simulink model "sim_DiscMRE_case1"  (R2024a)
settings: Solver=ode1  StartTime=0.0  StopTime=150  FixedStep=Ts  MaxStep=Ts  RelTol=1e-4
values from neighbouring files (symbols this model uses):
  x0 = x_init    [TO_sys.m]
undefined symbols (not defined in the file or in its folder): b0, b1, c1, c2, c3, curN, gamma, kpa, N, Phi0, th, Ts, vari, z0, zeta0
libraries: matrix_library x2
settings Model: Creator=stt  LastModifiedBy=stt
settings SolverCC: SolverResetMethod=Robust
settings OptimizationCC: ReuseModelBlockBuffer=off
settings RTWCC: GPUComputeCapability=3.5

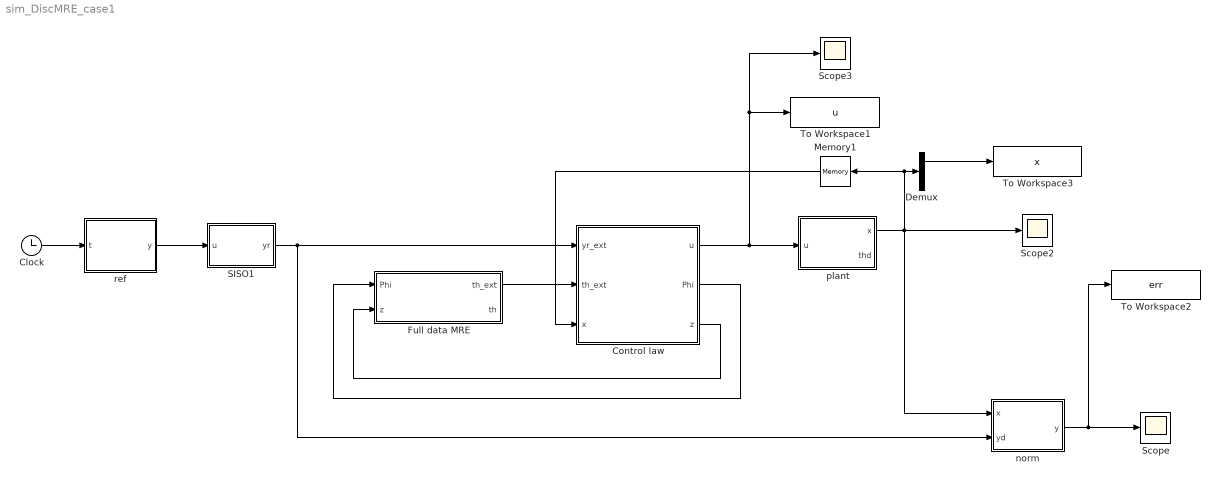
== system sim_DiscMRE_case1 ==
  Clock : Clock
  Control law : Subsystem
  Demux : Demux  Outputs=3
  Full data MRE : Subsystem
  Memory1 : Memory  InitialCondition=x0
  SISO1 : Subsystem
  Scope : Scope
  Scope2 : Scope
  Scope3 : Scope
  To Workspace1 : ToWorkspace  VariableName=u  SaveFormat=Timeseries  SampleTime=-1
  To Workspace2 : ToWorkspace  VariableName=err  SaveFormat=Timeseries  SampleTime=-1
  To Workspace3 : ToWorkspace  VariableName=x  SaveFormat=Timeseries  SampleTime=-1
  norm : MATLAB Function  TreatAsAtomicUnit=on
  plant : Subsystem
  ref : MATLAB Function  TreatAsAtomicUnit=on
  wires:
  SISO1/1(yr) -> norm/2(yd), Control law/1(yr_ext)
  norm/1(y) -> To Workspace2/1, Scope/1
  plant/1(x) -> Demux/1, Memory1/1, norm/1(x), Scope2/1
  Demux/1 -> To Workspace3/1
  Clock/1 -> ref/1(t)
  Control law/2(Phi) -> Full data MRE/1(Phi)
  Control law/1(u) -> To Workspace1/1, Scope3/1, plant/1(u)
  Memory1/1 -> Control law/3(x)
  Full data MRE/1(th_ext) -> Control law/2(th_ext)
  Control law/3(z) -> Full data MRE/2(z)
  ref/1(y) -> SISO1/1(u)

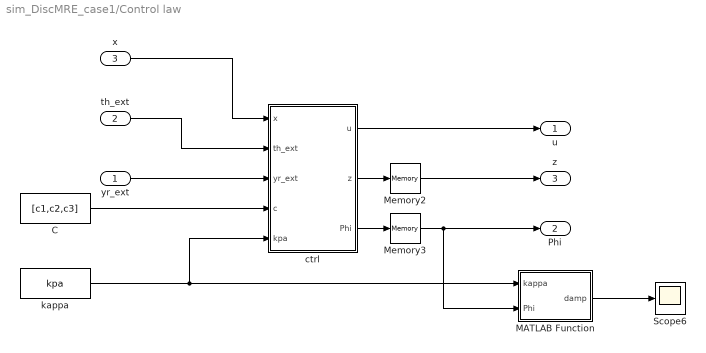
== system sim_DiscMRE_case1/Control law ==
  yr_ext : Inport
  th_ext : Inport  Port=2
  x : Inport  Port=3
  C : Constant  Value=[c1,c2,c3]
  MATLAB Function : MATLAB Function  TreatAsAtomicUnit=on
  Memory2 : Memory  InitialCondition=z0
  Memory3 : Memory  InitialCondition=Phi0
  Scope6 : Scope
  ctrl : MATLAB Function  TreatAsAtomicUnit=on
  kappa : Constant  Value=kpa
  u : Outport
  Phi : Outport  Port=2
  z : Outport  Port=3
  wires:
  ctrl/3(Phi) -> Memory3/1
  Memory3/1 -> MATLAB Function/2(Phi), Phi/1
  th_ext/1 -> ctrl/2(th_ext)
  kappa/1 -> ctrl/5(kpa), MATLAB Function/1(kappa)
  C/1 -> ctrl/4(c)
  Memory2/1 -> z/1
  ctrl/2(z) -> Memory2/1
  yr_ext/1 -> ctrl/3(yr_ext)
  x/1 -> ctrl/1(x)
  ctrl/1(u) -> u/1
  MATLAB Function/1(damp) -> Scope6/1

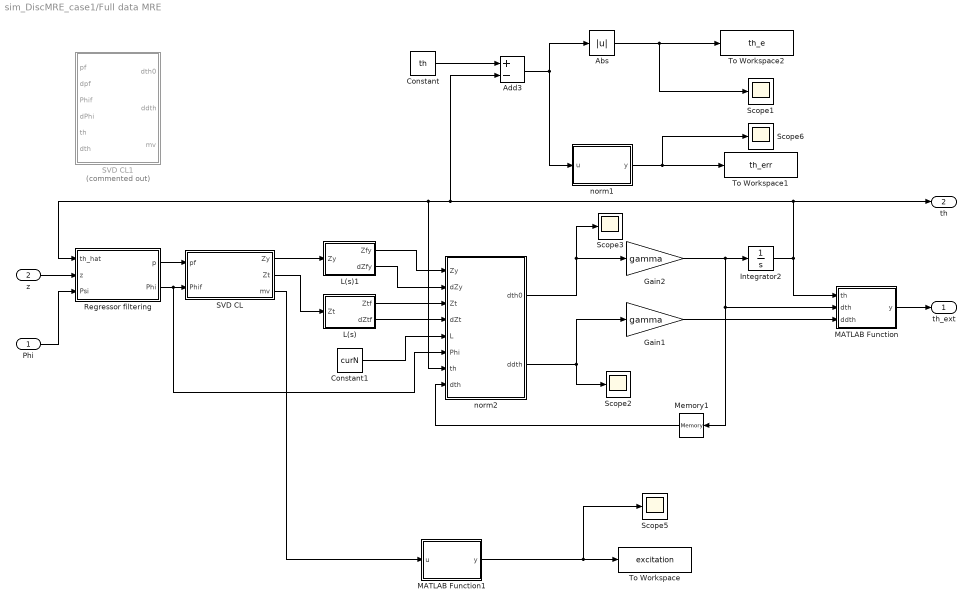
== system sim_DiscMRE_case1/Full data MRE ==
  Phi : Inport
  z : Inport  Port=2
  Abs : Abs  SaturateOnIntegerOverflow=off
  Add3 : Sum  Inputs=+-
  Constant : Constant  Value=th
  Constant1 : Constant  Value=curN
  Gain1 : Gain  Gain=gamma
  Gain2 : Gain  Gain=gamma
  Integrator2 : Integrator  InitialCondition=zeros(N,1)
  L(s) : Subsystem
  L(s)1 : Subsystem
  MATLAB Function : MATLAB Function  TreatAsAtomicUnit=on
  MATLAB Function1 : MATLAB Function  TreatAsAtomicUnit=on
  Memory1 : Memory  InitialCondition=zeros(N,1)
  Regressor filtering : Subsystem
  SVD CL : Subsystem
  SVD CL1 : Subsystem  Commented=on
  Scope{1..3,5..6} (5 alike) : Scope
  To Workspace : ToWorkspace  VariableName=excitation  SaveFormat=Timeseries  SampleTime=-1
  To Workspace1 : ToWorkspace  VariableName=th_err  SaveFormat=Timeseries  SampleTime=-1
  To Workspace2 : ToWorkspace  VariableName=th_e  SaveFormat=Timeseries  SampleTime=-1
  norm1 : MATLAB Function  TreatAsAtomicUnit=on
  norm2 : MATLAB Function  TreatAsAtomicUnit=on
  th_ext : Outport
  th : Outport  Port=2
  wires:
  MATLAB Function/1(y) -> th_ext/1
  MATLAB Function1/1(y) -> Scope5/1, To Workspace/1
  norm1/1(y) -> To Workspace1/1, Scope6/1
  Constant/1 -> Add3/1
  z/1 -> Regressor filtering/2(z)
  Phi/1 -> Regressor filtering/3(Psi)
  Gain1/1 -> MATLAB Function/3(ddth)
  Integrator2/1 -> MATLAB Function/1(th), th/1, norm2/7(th), Regressor filtering/1(th_hat), Add3/2
  Add3/1 -> norm1/1(u), Abs/1
  Abs/1 -> To Workspace2/1, Scope1/1
  Gain2/1 -> Memory1/1, MATLAB Function/2(dth), Integrator2/1
  Regressor filtering/1(p) -> SVD CL/1(pf)
  Regressor filtering/2(Phi) -> norm2/6(Phi), SVD CL/2(Phif)
  SVD CL/3(mv) -> MATLAB Function1/1(u)
  SVD CL/1(Zy) -> L(s)1/1(Zy)
  SVD CL/2(Zt) -> L(s)/1(Zt)
  L(s)1/1(Zfy) -> norm2/1(Zy)
  L(s)1/2(dZfy) -> norm2/2(dZy)
  L(s)/1(Ztf) -> norm2/3(Zt)
  L(s)/2(dZtf) -> norm2/4(dZt)
  Constant1/1 -> norm2/5(L)
  Memory1/1 -> norm2/8(dth)
  norm2/2(ddth) -> Gain1/1, Scope2/1
  norm2/1(dth0) -> Scope3/1, Gain2/1

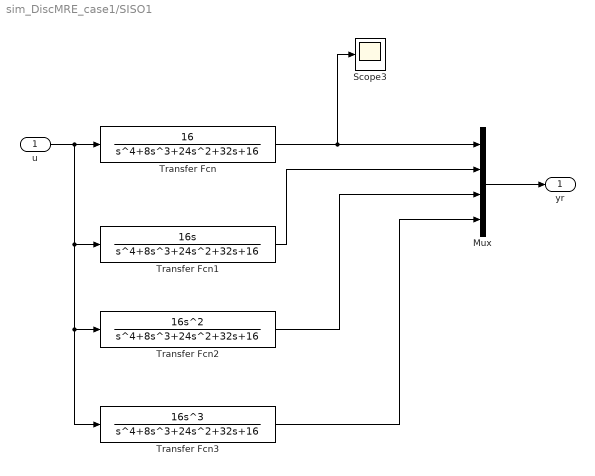
== system sim_DiscMRE_case1/SISO1 ==
  u : Inport
  Mux : Mux
  Scope3 : Scope
  Transfer Fcn : TransferFcn  Numerator=[16]  Denominator=[1 8 24 32 16]
  Transfer Fcn1 : TransferFcn  Numerator=[16 0]  Denominator=[1 8 24 32 16]
  Transfer Fcn2 : TransferFcn  Numerator=[16 0 0]  Denominator=[1 8 24 32 16]
  Transfer Fcn3 : TransferFcn  Numerator=[16 0 0 0]  Denominator=[1 8 24 32 16]
  yr : Outport
  wires:
  u/1 -> Transfer Fcn3/1, Transfer Fcn2/1, Transfer Fcn1/1, Transfer Fcn/1
  Transfer Fcn/1 -> Scope3/1, Mux/1
  Transfer Fcn1/1 -> Mux/2
  Transfer Fcn2/1 -> Mux/3
  Transfer Fcn3/1 -> Mux/4
  Mux/1 -> yr/1

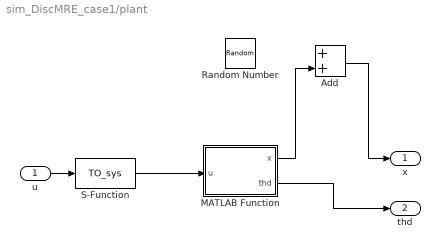
== system sim_DiscMRE_case1/plant ==
  u : Inport
  Add : Sum
  MATLAB Function : MATLAB Function  TreatAsAtomicUnit=on
  Random Number : RandomNumber  Variance=vari  SampleTime=Ts
  S-Function : S-Function  FunctionName=TO_sys  Parameters=x0,th  SFunctionDeploymentMode=off  EnableBusSupport=off
  x : Outport
  thd : Outport  Port=2
  wires:
  u/1 -> S-Function/1
  S-Function/1 -> MATLAB Function/1(u)
  Add/1 -> x/1
  MATLAB Function/2(thd) -> thd/1
  MATLAB Function/1(x) -> Add/2

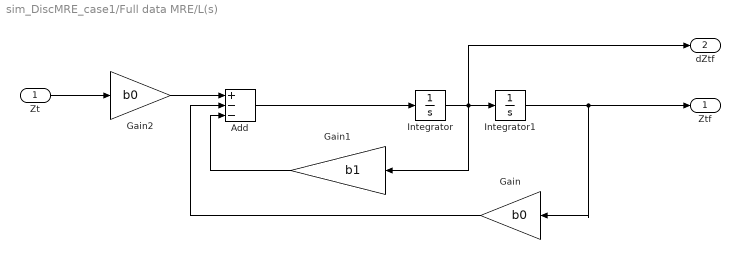
== system sim_DiscMRE_case1/Full data MRE/L(s) ==
  Zt : Inport
  Add : Sum  Inputs=+--
  Gain : Gain  Gain=b0
  Gain1 : Gain  Gain=b1
  Gain2 : Gain  Gain=b0
  Integrator : Integrator
  Integrator1 : Integrator
  Ztf : Outport
  dZtf : Outport  Port=2
  wires:
  Zt/1 -> Gain2/1
  Integrator1/1 -> Gain/1, Ztf/1
  Add/1 -> Integrator/1
  Integrator/1 -> Gain1/1, dZtf/1, Integrator1/1
  Gain1/1 -> Add/3
  Gain/1 -> Add/2
  Gain2/1 -> Add/1

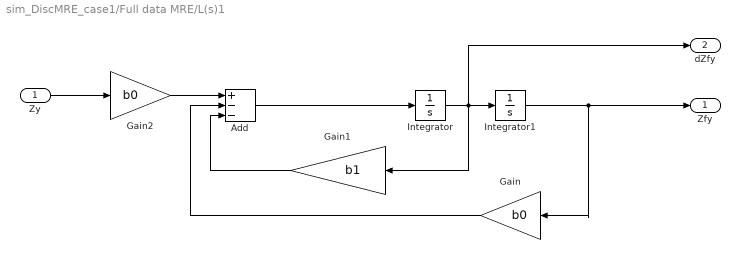
== system sim_DiscMRE_case1/Full data MRE/L(s)1 ==
  Zy : Inport
  Add : Sum  Inputs=+--
  Gain : Gain  Gain=b0
  Gain1 : Gain  Gain=b1
  Gain2 : Gain  Gain=b0
  Integrator : Integrator
  Integrator1 : Integrator
  Zfy : Outport
  dZfy : Outport  Port=2
  wires:
  Zy/1 -> Gain2/1
  Integrator1/1 -> Gain/1, Zfy/1
  Add/1 -> Integrator/1
  Integrator/1 -> Gain1/1, dZfy/1, Integrator1/1
  Gain1/1 -> Add/3
  Gain/1 -> Add/2
  Gain2/1 -> Add/1

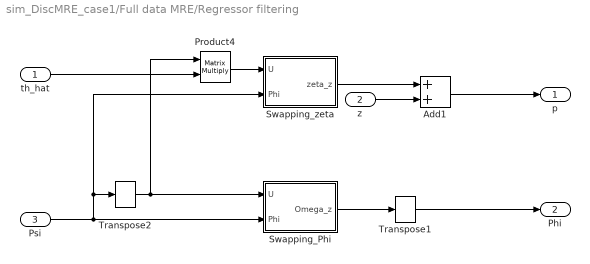
== system sim_DiscMRE_case1/Full data MRE/Regressor filtering ==
  th_hat : Inport
  z : Inport  Port=2
  Psi : Inport  Port=3
  Add1 : Sum
  Product4 : Product  Multiplication=Matrix(*)
  Swapping_Phi : Subsystem
  Swapping_zeta : Subsystem
  Transpose1 : matrix_library/Transpose
  Transpose2 : matrix_library/Transpose
  p : Outport
  Phi : Outport  Port=2
  wires:
  Product4/1 -> Swapping_zeta/1(U)
  th_hat/1 -> Product4/2
  Psi/1 -> Swapping_Phi/2(Phi), Swapping_zeta/2(Phi), Transpose2/1
  Swapping_zeta/1(zeta_z) -> Add1/1
  Transpose2/1 -> Swapping_Phi/1(U), Product4/1
  z/1 -> Add1/2
  Add1/1 -> p/1
  Swapping_Phi/1(Omega_z) -> Transpose1/1
  Transpose1/1 -> Phi/1

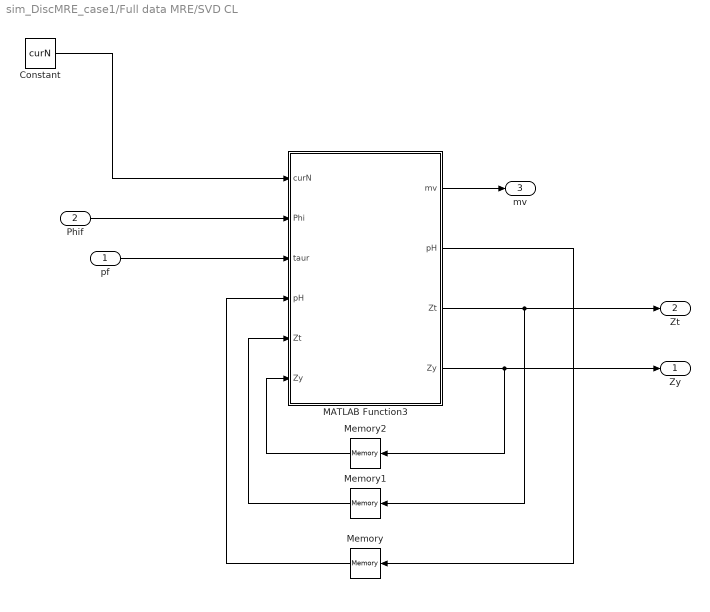
== system sim_DiscMRE_case1/Full data MRE/SVD CL ==
  pf : Inport
  Phif : Inport  Port=2
  Constant : Constant  Value=curN
  MATLAB Function3 : MATLAB Function  TreatAsAtomicUnit=on
  Memory : Memory
  Memory1 : Memory  InitialCondition=zeros(N,3*curN)
  Memory2 : Memory  InitialCondition=zeros(3*curN,1)
  Zy : Outport
  Zt : Outport  Port=2
  mv : Outport  Port=3
  wires:
  Memory/1 -> MATLAB Function3/4("pH ")
  pf/1 -> MATLAB Function3/3(taur)
  Memory1/1 -> MATLAB Function3/5("Zt ")
  Phif/1 -> MATLAB Function3/2(Phi)
  MATLAB Function3/3(Zt) -> Zt/1, Memory1/1
  MATLAB Function3/4(Zy) -> Zy/1, Memory2/1
  MATLAB Function3/2(pH) -> Memory/1
  Memory2/1 -> MATLAB Function3/6("Zy ")
  MATLAB Function3/1(mv) -> mv/1
  Constant/1 -> MATLAB Function3/1(curN)

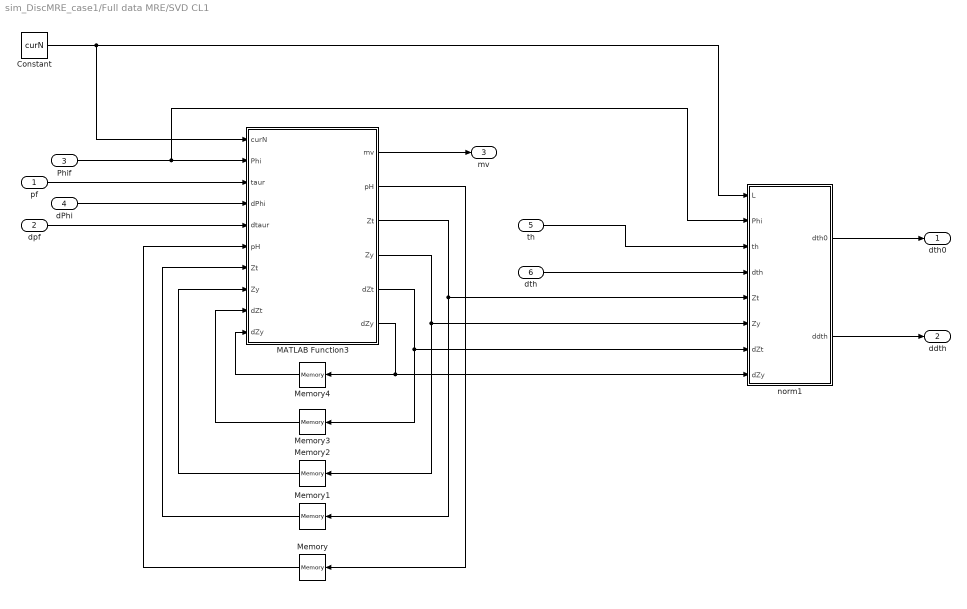
== system sim_DiscMRE_case1/Full data MRE/SVD CL1 ==
  pf : Inport
  dpf : Inport  Port=2
  Phif : Inport  Port=3
  dPhi : Inport  Port=4
  th : Inport  Port=5
  dth : Inport  Port=6
  Constant : Constant  Value=curN
  MATLAB Function3 : MATLAB Function  TreatAsAtomicUnit=on
  Memory : Memory
  Memory1 : Memory  InitialCondition=zeros(N,3*curN)
  Memory2 : Memory  InitialCondition=zeros(3*curN,1)
  Memory3 : Memory  InitialCondition=zeros(N,3*curN)
  Memory4 : Memory  InitialCondition=zeros(3*curN,1)
  norm1 : MATLAB Function  TreatAsAtomicUnit=on
  dth0 : Outport
  ddth : Outport  Port=2
  mv : Outport  Port=3
  wires:
  Memory/1 -> MATLAB Function3/6("pH ")
  pf/1 -> MATLAB Function3/3(taur)
  Memory1/1 -> MATLAB Function3/7("Zt ")
  Phif/1 -> norm1/2(Phi), MATLAB Function3/2(Phi)
  MATLAB Function3/3(Zt) -> Memory1/1, norm1/5(Zt)
  MATLAB Function3/4(Zy) -> Memory2/1, norm1/6(Zy)
  MATLAB Function3/2(pH) -> Memory/1
  Memory2/1 -> MATLAB Function3/8("Zy ")
  MATLAB Function3/1(mv) -> mv/1
  Constant/1 -> MATLAB Function3/1(curN), norm1/1(L)
  dPhi/1 -> MATLAB Function3/4(dPhi)
  dpf/1 -> MATLAB Function3/5(dtaur)
  Memory4/1 -> MATLAB Function3/10("dZy ")
  Memory3/1 -> MATLAB Function3/9("dZt ")
  MATLAB Function3/5(dZt) -> Memory3/1, norm1/7(dZt)
  MATLAB Function3/6(dZy) -> Memory4/1, norm1/8(dZy)
  th/1 -> norm1/3(th)
  dth/1 -> norm1/4(dth)
  norm1/2(ddth) -> ddth/1
  norm1/1(dth0) -> dth0/1

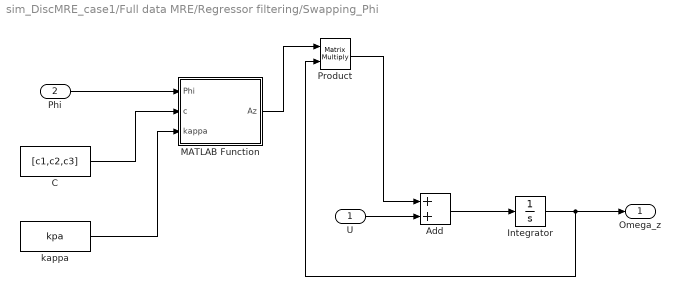
== system sim_DiscMRE_case1/Full data MRE/Regressor filtering/Swapping_Phi ==
  U : Inport
  Phi : Inport  Port=2
  Add : Sum
  C : Constant  Value=[c1,c2,c3]
  Integrator : Integrator
  MATLAB Function : MATLAB Function  TreatAsAtomicUnit=on
  Product : Product  Multiplication=Matrix(*)
  kappa : Constant  Value=kpa
  Omega_z : Outport
  wires:
  Phi/1 -> MATLAB Function/1(Phi)
  C/1 -> MATLAB Function/2(c)
  kappa/1 -> MATLAB Function/3(kappa)
  MATLAB Function/1(Az) -> Product/1
  Product/1 -> Add/1
  Add/1 -> Integrator/1
  U/1 -> Add/2
  Integrator/1 -> Product/2, Omega_z/1

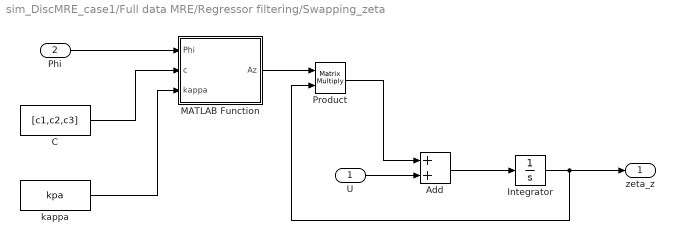
== system sim_DiscMRE_case1/Full data MRE/Regressor filtering/Swapping_zeta ==
  U : Inport
  Phi : Inport  Port=2
  Add : Sum
  C : Constant  Value=[c1,c2,c3]
  Integrator : Integrator  InitialCondition=zeta0
  MATLAB Function : MATLAB Function  TreatAsAtomicUnit=on
  Product : Product  Multiplication=Matrix(*)
  kappa : Constant  Value=kpa
  zeta_z : Outport
  wires:
  Phi/1 -> MATLAB Function/1(Phi)
  C/1 -> MATLAB Function/2(c)
  kappa/1 -> MATLAB Function/3(kappa)
  MATLAB Function/1(Az) -> Product/1
  Product/1 -> Add/1
  Add/1 -> Integrator/1
  U/1 -> Add/2
  Integrator/1 -> Product/2, zeta_z/1

== matlab function sim_DiscMRE_case1/Full data MRE/norm1 ==
  data: u input; y output
function y = fcn(u)

y = norm(u);

== matlab function sim_DiscMRE_case1/Full data MRE/SVD CL/MATLAB Function3 ==
  data: curN input; mv output; pH output; Zt output; Zy output; Phi input; taur input; pH input; Zt input; Zy input
function [mv,pH,Zt,Zy] = fcn(curN,Phi,taur,pH,Zt,Zy)

[N,n]=size(Phi);
L=curN;

if pH<L
    pH=pH+1;
    Zt(:,n*(pH-1)+1:pH*n)=Phi;
    Zy(n*(pH-1)+1:pH*n)=taur;
    S_old=min(svd(Zt));
else
    T=Zt;
    S_old=min(svd(Zt));
    S=zeros(L,1);
    for j=1:pH
        Zt(:,n*(j-1)+1:j*n)=Phi;
        S(j)=min(svd(Zt));
        Zt=T;
    end
    ind=find(max(S)==S);
    if max(S)>S_old && min(S)>1e-4
        j0=ind(1);
        Zt(:,n*(j0-1)+1:j0*n)=Phi;
        Zy(n*(j0-1)+1:j0*n)=taur;
        S_old=max(S);
    end
end

mv=S_old;

== matlab function sim_DiscMRE_case1/Full data MRE/norm2 ==
  data: Zy input; dZy input; Zt input; dZt input; dth0 output; L input; Phi input; th input; dth input; ddth output
function [dth0,ddth] = fcn(Zy,dZy,Zt,dZt,L,Phi,th,dth)


[N,n]=size(Phi);
ddth=zeros(N,1);
dth0=zeros(N,1);

for k=1:L
    d1=dZt(:,n*(k-1)+1:k*n)*(Zy(n*(k-1)+1:k*n)-Zt(:,n*(k-1)+1:k*n)'*th);
    d2=Zt(:,n*(k-1)+1:k*n)*(dZy(n*(k-1)+1:k*n)-dZt(:,n*(k-1)+1:k*n)'*th-Zt(:,n*(k-1)+1:k*n)'*dth);
    % d1=dZt(:,n*(k-1)+1:k*n)*(Zt(:,n*(k-1)+1:k*n)'*thd-Zt(:,n*(k-1)+1:k*n)'*th);
    % d2=Zt(:,n*(k-1)+1:k*n)*(dZt(:,n*(k-1)+1:k*n)'*thd-dZt(:,n*(k-1)+1:k*n)'*th-Zt(:,n*(k-1)+1:k*n)'*dth);
    ddth=ddth+d1+d2;
    dth0=dth0+Zt(:,n*(k-1)+1:k*n)*(Zy(n*(k-1)+1:k*n)-Zt(:,n*(k-1)+1:k*n)'*th);
end
% ddth=dZt*(Zy'-Zt'*th)+Zt*(dZy'-dZt'*th-Zt'*dth);
% ddth=ddth/10;
% dth0=dth0/10;

== matlab function sim_DiscMRE_case1/Full data MRE/SVD CL1/MATLAB Function3 ==
  data: curN input; mv output; pH output; Zt output; Zy output; dZt output; dZy output; Phi input; taur input; dPhi input; dtaur input; pH input; Zt input; Zy input; dZt input; dZy input
function [mv,pH,Zt,Zy,dZt,dZy] = fcn(curN,Phi,taur,dPhi,dtaur,pH,Zt,Zy,dZt,dZy)

[N,n]=size(Phi);
L=curN;

if pH<L
    pH=pH+1;
    Zt(:,n*(pH-1)+1:pH*n)=Phi;
    Zy(n*(pH-1)+1:pH*n)=taur;
    dZt(:,n*(pH-1)+1:pH*n)=dPhi;
    dZy(n*(pH-1)+1:pH*n)=dtaur;
    S_old=min(svd(Zt));
else
    T=Zt;
    S_old=min(svd(Zt));
    S=zeros(L,1);
    for j=1:pH
        Zt(:,n*(j-1)+1:j*n)=Phi;
        S(j)=min(svd(Zt));
        Zt=T;
    end
    ind=find(max(S)==S);
    if max(S)>S_old && min(S)>1e-4
        j0=ind(1);
        Zt(:,n*(j0-1)+1:j0*n)=Phi;
        Zy(n*(j0-1)+1:j0*n)=taur;
        dZt(:,n*(j0-1)+1:j0*n)=dPhi;
        dZy(n*(j0-1)+1:j0*n)=dtaur;
        S_old=max(S);
    end
end

mv=S_old;

== matlab function sim_DiscMRE_case1/Control law/MATLAB Function ==
  data: kappa input; damp output; Phi input
function damp = fcn(kappa,Phi)
kap1=kappa(1);kap2=kappa(2);kap3=kappa(3);
phi1=Phi(:,1);phi2=Phi(:,2);phi3=Phi(:,3);
damp=-[kap1*norm(phi1)^2,kap2*norm(phi2)^2,kap3*norm(phi3)^2];

== matlab function sim_DiscMRE_case1/Full data MRE/SVD CL1/norm1 ==
  data: dth0 output; L input; Phi input; th input; dth input; Zt input; ddth output; Zy input; dZt input; dZy input
function [dth0,ddth] = fcn(L,Phi,th,dth,Zt,Zy,dZt,dZy)


[N,n]=size(Phi);
ddth=zeros(N,1);
dth0=zeros(N,1);
thd=[0.4,0.5,0.1]';

for k=1:L
    d1=dZt(:,n*(k-1)+1:k*n)*(Zy(n*(k-1)+1:k*n)-Zt(:,n*(k-1)+1:k*n)'*th);
    d2=Zt(:,n*(k-1)+1:k*n)*(dZy(n*(k-1)+1:k*n)-dZt(:,n*(k-1)+1:k*n)'*th-Zt(:,n*(k-1)+1:k*n)'*dth);
    % d1=dZt(:,n*(k-1)+1:k*n)*(Zt(:,n*(k-1)+1:k*n)'*thd-Zt(:,n*(k-1)+1:k*n)'*th);
    % d2=Zt(:,n*(k-1)+1:k*n)*(dZt(:,n*(k-1)+1:k*n)'*thd-dZt(:,n*(k-1)+1:k*n)'*th-Zt(:,n*(k-1)+1:k*n)'*dth);
    ddth=ddth+d1+d2;
    dth0=dth0+Zt(:,n*(k-1)+1:k*n)*(Zy(n*(k-1)+1:k*n)-Zt(:,n*(k-1)+1:k*n)'*th);
end
% ddth=dZt*(Zy'-Zt'*th)+Zt*(dZy'-dZt'*th-Zt'*dth);
% ddth=ddth/10;
% dth0=dth0/10;

== matlab function sim_DiscMRE_case1/Control law/ctrl ==
  data: x input; th_ext input; yr_ext input; u output; c input; kpa input; z output; Phi output
function [u,z,Phi] = fcn(x,th_ext,yr_ext,c,kpa)



[alpha1,alpha2,u,z,Phi]=virtual_ctrl(x,th_ext,yr_ext,kpa,c);
vir_u=[alpha1,alpha2];

== matlab function sim_DiscMRE_case1/Full data MRE/MATLAB Function1 ==
  data: u input; y output
function y = fcn(u)

y = min(svd(u));

== matlab function sim_DiscMRE_case1/ref ==
  data: t input; y output
function y = fcn(t)


if t<50
    y=-0.25;
% elseif t<80
    % y=-0.5;
elseif t<100
    y=-1;
else
    y=0;
end
% A=1;T=1;
% y=[A*sin(T*t);A*T*cos(T*t);-A*T*T*sin(T*t);-A*T*T*T*cos(T*t)];
% y=1.2*sin(0.8*t)+0.8*cos(0.4*t)-0.8;

== matlab function sim_DiscMRE_case1/norm ==
  data: x input; y output; yd input
function y= fcn(x,yd)
err=x(1)-yd(1);
y = abs(err);

== matlab function sim_DiscMRE_case1/Full data MRE/Regressor filtering/Swapping_zeta/MATLAB Function ==
  data: Phi input; Az output; c input; kappa input
function Az = fcn(Phi,c,kappa)
c1=c(1);c2=c(2);c3=c(3);
kap1=kappa(1);kap2=kappa(2);kap3=kappa(3);
phi1=Phi(:,1);phi2=Phi(:,2);phi3=Phi(:,3);
Dg=-[c1+kap1*norm(phi1)^2,c2+kap2*norm(phi2)^2,c3+kap3*norm(phi3)^2];
Az=diag(Dg)+diag([1,1],1)-diag([1,1],-1);

== matlab function sim_DiscMRE_case1/Full data MRE/Regressor filtering/Swapping_Phi/MATLAB Function ==
  data: Phi input; Az output; c input; kappa input
function Az = fcn(Phi,c,kappa)
c1=c(1);c2=c(2);c3=c(3);
kap1=kappa(1);kap2=kappa(2);kap3=kappa(3);
phi1=Phi(:,1);phi2=Phi(:,2);phi3=Phi(:,3);
Dg=-[c1+kap1*norm(phi1)^2,c2+kap2*norm(phi2)^2,c3+kap3*norm(phi3)^2];
Az=diag(Dg)+diag([1,1],1)-diag([1,1],-1);

== matlab function sim_DiscMRE_case1/plant/MATLAB Function ==
  data: u input; x output; thd output
function [x,thd] = fcn(u)

x=u(1:3);
thd=u(4:6);

== matlab function sim_DiscMRE_case1/Full data MRE/MATLAB Function ==
  data: th input; y output; dth input; ddth input
function y = fcn(th,dth,ddth)

y = [th,dth,ddth];
